simulink subsystem "TheSecondSubmodel"  (R2023a)
settings: Solver=VariableStepAuto  StartTime=0.0  StopTime=10.0  RelTol=1e-3
undefined symbols (not defined in the file): ProjectForLab5
settings Model: Creator=79056  LastModifiedBy=79056

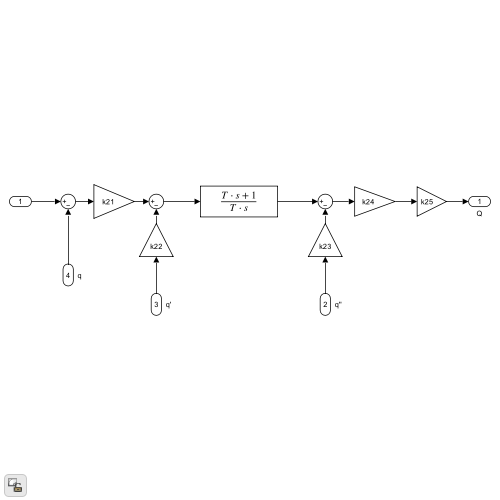
[thumbnail: Simulink's stored preview of the top-level diagram]
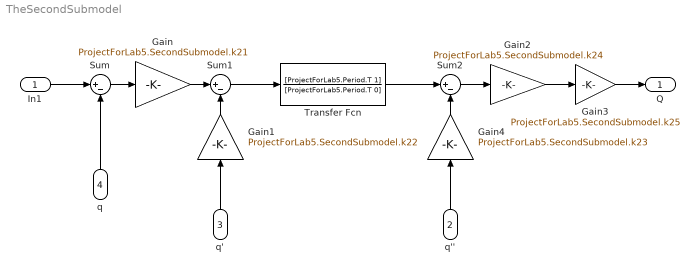
== system TheSecondSubmodel ==
  In1 : Inport
  q'' : Inport  Port=2
  q' : Inport  Port=3
  q : Inport  Port=4
  Gain : Gain  Gain=ProjectForLab5.SecondSubmodel.k21
  Gain1 : Gain  Gain=ProjectForLab5.SecondSubmodel.k22
  Gain2 : Gain  Gain=ProjectForLab5.SecondSubmodel.k24
  Gain3 : Gain  Gain=ProjectForLab5.SecondSubmodel.k25
  Gain4 : Gain  Gain=ProjectForLab5.SecondSubmodel.k23
  Sum : Sum  Inputs=|+-
  Sum1 : Sum  Inputs=|+-
  Sum2 : Sum  Inputs=|+-
  Transfer Fcn : TransferFcn  Numerator=[ProjectForLab5.Period.T 1]  Denominator=[ProjectForLab5.Period.T 0]
  Q : Outport
  wires:
  In1/1 -> Sum/1
  Sum/1 -> Gain/1
  Gain/1 -> Sum1/1
  Gain1/1 -> Sum1/2
  Sum1/1 -> Transfer Fcn/1
  Transfer Fcn/1 -> Sum2/1
  Sum2/1 -> Gain2/1
  Gain2/1 -> Gain3/1
  Gain4/1 -> Sum2/2
  Gain3/1 -> Q/1
  q''/1 -> Gain4/1
  q'/1 -> Gain1/1
  q/1 -> Sum/2
